simulink model "ad9361_rx_fastattack"  (R2017b)
settings: Solver=ode23  StartTime=0.0  StopTime=inf  RelTol=1e-3  EnableMultiTasking=on
PreLoadFcn:
  | SampleTime_rx = 6.51041666666666667e-8;
  | 
  | adi9361_preload(bdroot,'rx')
undefined symbols (not defined in the file or in its folder): D, dBval, DCLeak_Matrix, fuzz_val, GainImb_Matrix, IP2_Matrix, IP3_Matrix, magnitude, var
libraries: simrfV2elements x13, dsparch4 x8, dspsrcs4 x8, dspmathops x6, dspmlti4 x5, simulink x5, simrfV2util1 x4, fl_lib x4, simrfV2junction1 x3, simulink_extras x2, dspsigattribs x2, simrfV2sources1 x2
(part 1 of 2)
CloseFcn:
  | clear ad9361_rx_hm1Filt ad9361_rx_hm2Filt;
  | clear ad9361_rx_hm3Filt ad9361_rx_hm4Filt;
  | clear SampleTime_rx;
settings Model: SimulationMode=accelerator  Creator=The MathWorks Inc.  LastModifiedBy=ppradhan
settings DataIOCC: ExternalInput=txWaveform  SaveFormat=StructureWithTime  SaveOutput=off  SignalLogging=off  DSMLogging=off  SaveTime=off  OutputSaveName=rx
settings OptimizationCC: DefaultParameterBehavior=Inlined  InlineInvariantSignals=on  EfficientMapNaN2IntZero=off  LifeSpan=inf  SimCompilerOptimization=on
settings DebuggingCC: ReadBeforeWriteMsg=DisableAll  WriteAfterWriteMsg=DisableAll  WriteAfterReadMsg=DisableAll  UnderspecifiedInitializationDetection=Classic  MergeDetectMultiDrivingBlocksExec=none  SolverPrmCheckMsg=warning  InheritedTsInSrcMsg=none  MultiTaskDSMMsg=none  IntegerOverflowMsg=none  AllowSymbolicDim=off  SFUnexpectedBacktrackingDiag=warning  SFNoUnconditionalDefaultTransitionDiag=none  SFUndirectedBroadcastEventsDiag=none  SFExecutionAtInitializationDiag=none  IntegerSaturationMsg=none
settings HardwareCC: ProdBitPerPointer=32  ProdBitPerSizeT=32  ProdBitPerPtrDiffT=32  ProdLargestAtomicFloat=None  ProdIntDivRoundTo=Undefined  ProdEndianess=Unspecified  ProdWordSize=32  ProdHWDeviceType=32-bit Generic  TargetBitPerPointer=64  TargetBitPerSizeT=64  TargetBitPerPtrDiffT=64  TargetLongLongMode=on  TargetIntDivRoundTo=Zero  TargetEndianess=LittleEndian  TargetWordSize=64  TargetHWDeviceType=MATLAB Host  ProdEqTarget=off
settings ModelReferenceCC: UpdateModelReferenceTargets=IfOutOfDate  PropagateSignalLabelsOutOfModel=off
settings SFSimCC: SFSimEcho=off
settings CodeAppCC: MaxIdLength=128  StateflowObjectComments=on
settings GRTTargetCC: TargetLangStandard=C89/C90 (ANSI)  GeneratePreprocessorConditionals=Disable all  CombineOutputUpdateFcns=off  GRTInterface=on
settings ConfigComp: CovMetricSettings=dw  CovHtmlReporting=on  CovSaveCumulativeToWorkspaceVar=on  CovSaveSingleToWorkspaceVar=on  CovExternalEMLEnable=off  CovSFcnEnable=off
settings SimscapeCC: ExplicitSolverDiagnosticOptions=none

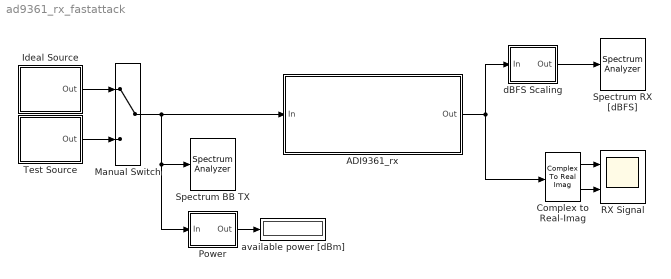
== system ad9361_rx_fastattack ==
  ADI9361_rx : Subsystem  mask(ADI9361_RX){TestSignal=20MHz LTE, LOFreq=2.1e9, Trf=SampleTime_rx/1.5}
      mask prompts: TestSignal "Filter Configuration:"; LOFreq "LO Frequency [Hz]:"; Trf "Step Size RF Simulation [s]:"
      mask help: Model an Analog Devices AD9361 RF Receiver.
      mask init:
      | load ADI9361Tables;
      | ad9361_rx_pars = ad9361_rx_initfcn(gcb,'Init');
      | assignin('base', 'ad9361_rx_hm1Filt', ad9361_rx_pars.ad9361_rx_hm1Filt);
      | assignin('base', 'ad9361_rx_hm2Filt', ad9361_rx_pars.ad9361_rx_hm2Filt);
      | assignin('base', 'ad9361_rx_hm3Filt', ad9361_rx_pars.ad9361_rx_hm3Filt);
      | assignin('base', 'ad9361_rx_hm4Filt', ad9361_rx_pars.ad9361_rx_hm4Filt);
      mask Help:
      | Model an Analog Devices AD9361 RF Receiver. This model predicts thermal noise, spectral growth, LO carrier leakage and image signals, quantization noise in manual and slow attack control mode.
      | 
      | To change the automatic gain control mode, toggle the manual switch between manual mode and slow-attack control mode under the receiver mask. For manual mode, directly specify the index of the gain table in the constant block "manual index".
      | 
      | For signals with LTE 5MHz, LTE 10 MHz and LTE 20 MHz characteristics, the default configurations recommended by Analog Devices are directly available.
      | 
      | The filters are programmable. Use the Analog Devices Wizard App to custom design Filters. Select the option Custom in the Filter Configuration menu and click Design Filter button. The Filter Design app will open automatically. Make sure a receiver filter is designed instead of a transmitter filter. After designing the filter, click the button Export to Workspace in the App. The custom filter design is saved in the model set up. Next time a simulation is setup with custom filter configuration, the latest filter design is used.
      | 
      | Make sure that the input signal sample time and the expected step size of the RF simulation are the same. In case of a mismatch, an error is generated.
      mask TypeOptions TestSignal: 5MHz LTE | 10MHz LTE | 20MHz LTE | Custom
      mask Callback TestSignal:
      | % Set Mask visibilites and enables
      | ad9361_rx_mask_callbacks(gcb,'TestSignal')
      mask DialogControl Control2 Prompt: SpacerDesign
      mask DialogControl DesignFilter Prompt: Design Filter
      mask DialogControl DesignFilter Callback: ad9361_rx_initfcn(gcb,'DesignFilter');
      mask Display: text(0.5,0.5,'AD9361_RX','horizontalAlignment','center');
  Complex to Real-Imag : ComplexToRealImag
  Ideal Source : Subsystem  mask{Sel=Single CW tone, CW=2e6, Pow=-60, Tstep=3.255208333333334e-08, Ovs=1.5}
      mask prompts: Sel "Select source"; CW "Frequency (Hz)"; Pow "Power (dBm)"; Tstep "Sample time (s)"; Ovs "Oversampling"
      mask TypeOptions Sel: CW + 1MHz tone | Single CW tone | Dual CW tone
      mask DialogControl DescGroupVar Prompt: Ideal Test Source
  Manual Switch : ManualSwitch
  "Power  " : Subsystem  mask{R=50}
      mask prompts: R "Reference Impedance [Ohm]"
      mask DialogControl DescGroupVar Prompt: Power Meter
  RX Signal : Scope  NumInputPorts=2
  Spectrum BB TX : SpectrumAnalyzer
  Spectrum RX [dBFS] : SpectrumAnalyzer
  Test Source : Subsystem  mask{TestSigType=20MHz LTE-like test signal, RxCustVector=complex(rand(1000,1), rand(1000,1)), Tstep=3.255208333333334e-08, OverSample=1.5, LTE_Pow=-50, hasBlockerCW=off, CW_Blocker_Freq=3e6, CW_Blocker_Pow=-20, hasBlockerLTE=off, LTE_Blocker_OffsetFreq=3e6, LTE_Blocker_Pow=-30}
      mask prompts: TestSigType "Test signal"; RxCustVector "Custom test vector complex data (I, Q)"; Tstep "Sample time (s)"; OverSample "Oversampling"; LTE_Pow "Power (dBm)"; hasBlockerCW "CW blocker"; CW_Blocker_Freq "Frequency CW blocker (Hz)"; CW_Blocker_Pow "Power CW blocker (dBm)"; hasBlockerLTE "LTE-like blocker"; LTE_Blocker_OffsetFreq "Frequency offset LTE-like blocker (Hz)"; LTE_Blocker_Pow "Power LTE-like blocker (dBm)"
      mask init:
      | load LTE_data;
      | load LTE_blocker;
      | 
      | if strcmpi(TestSigType,'5MHz LTE-like test signal')
      |     tx = tx5;
      |     tx_bl = tx5_bl;
      |     SampleTime_rx = 1/info5.SamplingRate;
      |     LTE = 5;
      | elseif strcmpi(TestSigType,'10MHz LTE-like test signal')
      |     tx = tx10;
      |     tx_bl = tx10_bl;
      |     LTE = 10;
      |     SampleTime_rx = 1/info10.SamplingRate;
      | elseif strcmpi(TestSigType,'20MHz LTE-like test signal')
      |     tx = tx20;
      |     tx_bl = tx20_bl;
      |     LTE = 20;
      |     SampleTime_rx = 1/info20.SamplingRate;
      | elseif strcmpi(TestSigType,'Custom Signal (LTE blocker NOT allowed)')
      |     LTE = 0;
      |     tx = RxCustVector;
      |     tx_bl = RxCustVector;
      |     SampleTime_rx = str2num(get_param(gcb,'Tstep'));
      | else
      |     error(message('simrf:simrfad9361:UnknownTestSig',gcb,TestSigType));
      | end
      | if ~strcmp(TestSigType,'Custom signal (LTE blocker NOT allowed)')
      |     assignin('base', 'SampleTime_rx', SampleTime_rx);
      | end
      | if ~any(strcmpi(get_param(bdroot(gcb), 'SimulationStatus'),             ...
      |         {'running' 'paused'}))
      |     set_param(gcb,'Tstep',num2str(SampleTime_rx,16));
      |     idlSrc = [bdroot '/Ideal Source'];
      |     set_param(idlSrc,'Tstep',num2str(SampleTime_rx,16));
      |     p = Simulink.Mask.get(gcb);
      |     p.Parameters(3).Value = num2str(SampleTime_rx,16);
      | end
      mask TypeOptions TestSigType: 5MHz LTE-like test signal | 10MHz LTE-like test signal | 20MHz LTE-like test signal | Custom Signal (LTE blocker NOT allowed)
      mask Callback TestSigType:
      | % Set Mask visibilites and enables
      | ad9361_rx_mask_callbacks(gcb,'TestSigType')
      mask Callback hasBlockerCW:
      | % Set Mask visibilites and enables
      | ad9361_rx_mask_callbacks(gcb,'hasBlockerCW')
      mask Callback hasBlockerLTE:
      | % Set Mask visibilites and enables
      | ad9361_rx_mask_callbacks(gcb,'hasBlockerLTE')
      mask DialogControl DescGroupVar Prompt: Test Source RX
  available power [dBm] : Display
  dBFS Scaling : Subsystem
  wires:
  Test Source/1(Out) -> Manual Switch/2
  Ideal Source/1(Out) -> Manual Switch/1
  Manual Switch/1 -> Spectrum BB TX/1, "Power  "/1(In), ADI9361_rx/1(In)
  "Power  "/1(Out) -> available power [dBm]/1
  dBFS Scaling/1(Out) -> Spectrum RX [dBFS]/1
  ADI9361_rx/1(Out) -> Complex to Real-Imag/1, dBFS Scaling/1(In)
  Complex to Real-Imag/1 -> RX Signal/1
  Complex to Real-Imag/2 -> RX Signal/2

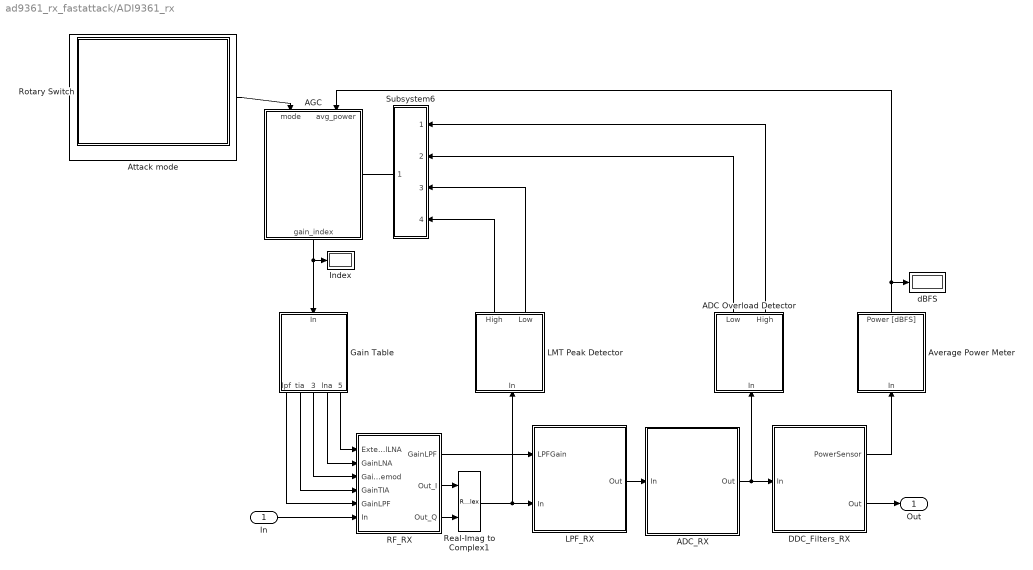
== system ad9361_rx_fastattack/ADI9361_rx ==
  In : Inport
  ADC Overload Detector : Subsystem  mask{Ncycles=4, Lthreshold=47, Hthreshold=58}
      mask prompts: Ncycles "Number of Integration Cycles"; Lthreshold "Low Threshold"; Hthreshold "High Threshold"
      mask DialogControl DescGroupVar Prompt: ADC Overload Detector
  ADC_RX : Subsystem
  AGC : Stateflow chart  TreatAsAtomicUnit=on  mask{T=1, PeakOverLoadWait=1, SettlingDelay=32, FIR_Ts=ad9361_rx_pars.Tadc*ad9361_rx_pars.HB_interp, LMT_G_dec_fast=2, ADC_G_dec_fast=2, AGC_G_dec_fast=1, AGC_G_dec_slow=1, AGC_G_inc_fast=1, AGC_G_inc_slow=1, ManualGainIndex=76, C=61440 %approx 1ms, N_LMT_H=10, N_LMT_L=10, N_ADC_H=10, N_ADC_L=10, PT_HH=-8, PT_H=-10, PT_L=-12, PT_LL=-15, AGC_lock_level=-10, Max_Increase=5, EnableIncrGain=1, EnableGainIncAfterLock=1, AGC_attack_delay=10, EnergyDetectCount=32, IncrTime=5, LowPower=-13, PostLockStepSize=1, PowerMeasDuration=64, GainReset=Max Gain, GainOffset=5, EnergyLost=1, StrongerSignalThreshold=10, GainLockExitCount=8, Overrange=8}
      mask prompts: T "Extra delay margin [us]"; PeakOverLoadWait "Peak Overload Wait Time [cycles]"; SettlingDelay "Settling Delay Power Meter [cycles]"; FIR_Ts "FIR Input Clock Time"; LMT_G_dec_fast "LMT peak large decrement"; ADC_G_dec_fast "ADC peak large decrement"; AGC_G_dec_fast "Average Power large decrement"; AGC_G_dec_slow "Average Power small decrement"; AGC_G_inc_fast "Average Power large increment"; AGC_G_inc_slow "Average Power small increment"; ManualGainIndex "Gain Index"; C "Gain Update Counter [cycles]"; N_LMT_H "LMT Upper Count"; N_LMT_L "LMT Lower Count"; N_ADC_H "ADC Upper Count"; N_ADC_L "ADC Lower Count"; PT_HH "Outer Threshold High [dBFS]"; PT_H "Inner Threshold High [dBFS]"; PT_L "Inner Threshold Low [dBFS]"; PT_LL "Outer Threshold Low [dBFS]"; AGC_lock_level "AGC Lock Level [dBFS]"; Max_Increase "AGC Lock Level Max Increase [Index]"; EnableIncrGain "Enable Gain Increment [0/1]"; EnableGainIncAfterLock "Enable Gain Increment After Gain Lock [0/1]"; AGC_attack_delay "Attack delay [us]"; EnergyDetectCount "Energy Detect Count [cycles]"; IncrTime "Increment Time [cycles]"; LowPower "Low Power Threshold"; PostLockStepSize "Post Lock Level Step Size [Index]"; PowerMeasDuration "Power Measurement Duration - State 5 [cycles]"; GainReset "Gain Index When Reset"; GainOffset "Optimize Gain Offset"; EnergyLost "Energy Lost Level [dB]"; StrongerSignalThreshold "Stronger Signal Threshold [dB]"; GainLockExitCount "Gain Lock Exit Count [cycles]"; Overrange "Overrange Count [Events]"
      mask init:
      | EnergyDetectCount = EnergyDetectCount*FIR_Ts;
      | C = C*FIR_Ts;
      | SettlingDelay = SettlingDelay*FIR_Ts;
      | PeakOverLoadWait = PeakOverLoadWait*FIR_Ts;
      | PowerMeasDuration = PowerMeasDuration*FIR_Ts;
      | IncrTime = IncrTime*FIR_Ts;
      | 
      | tmp = get_param(gcb,'parent');
      | n = get_param([tmp, '/Average Power Meter'], 'Ncycles');
      | DecPowerMeasDuration = str2num(n)*FIR_Ts;
  Attack mode : Constant  Value=0  SampleTime=-1
  Average Power Meter : Subsystem  mask{Ncycles=64}
      mask prompts: Ncycles "Number of Integration Cycles"
      mask DialogControl DescGroupVar Prompt: Average Power Meter
  DDC_Filters_RX : Subsystem
  Gain Table : Subsystem
  "Index " : Display
  LMT Peak Detector : Subsystem  mask{HThreshold=800, LThreshold=704}
      mask prompts: HThreshold "High Threshold [mV]"; LThreshold "Low Threshold [mV]"
      mask DialogControl DescGroupVar Prompt: LMT Peak Detector
  LPF_RX : Subsystem
  RF_RX : Subsystem  mask{RF=LOFreq, Tstep=Trf, Imp=on}
      mask prompts: RF "Center Frequency [Hz]"; Tstep "Sample Time [s]"; Imp "RF Impairments [on/off]"
      mask init:
      | freq = [0.8e9, 2.4e9, 5.5e9];
      | nf   = [2,       3,        3.8];
      | NF   = interp1(freq, nf, RF);
      | 
      | index_gain3  = [6,  16, 20, 23, 28,  30,  33, 34, 36, 37, 54, 55,  73,  76];
      | iip3_800MHz  = [10, 10, 10, 8,   8,   10,  9,   -3, -5, -5, -8, -13, -14, -18];
      | iip3_2p4GHz  = [9,  9,   9,   8,   7,    9,   8,   0,   0,  -5, -5, -7,   -8,   -10];
      | iip3_5p5GHz  = [16,10, 10, 11,  11, 11, 11,  11, 11, -3, -6, -7,  -10, -16];
      | 
      | index_gain2  = [20, 36, 68, 76];
      | iip2_800MHz  = [80, 80, 58, 48];
      | iip2_2p4GHz  = [70, 70, 60, 50];
      | iip2_5p5GHz  = [70, 70, 60, 45];
      | 
      | if RF<=1.3e9
      |     ind_lna = (0:3);
      |     lna_gain = [5, 17, 19 24];
      |     ind_mixer = (0:15);
      |     mixer_gain = [0, 3, 9, (2:14)+11];
      |     ind_tia = (0:1);
      |     tia_gain = [-6, 0];
      |     IIP3 = iip3_800MHz;
      |     IIP2 = iip2_800MHz;
      | elseif RF <= 4e9
      |     ind_lna = (0:3);
      |     lna_gain = [3, 14, 17, 21];
      |     ind_mixer = (0:15);
      |     mixer_gain = [0, 3, 9, (3:15)+11];
      |     ind_tia = (0:1);
      |     tia_gain = [-6, 0];
      |     IIP3 = iip3_2p4GHz;
      |     IIP2 = iip2_2p4GHz;
      | else
      |     ind_lna = (0:3);
      |     lna_gain = [-4, 10, 13, 14];
      |     ind_mixer = (0:15);
      |     mixer_gain = [0, 3, 8, (1:13)+11];
      |     ind_tia = (0:1);
      |     tia_gain = [-6, 0];
      |     IIP3 = iip3_5p5GHz;
      |     IIP2 = iip2_5p5GHz;
      | end
      | %index = [0 16 26 36 46 56 66 76];
      | index  = [0 6 15 26 37 48 58 69 76];
      | if Imp == 0
      |     NF = 0;
      |     IIP3 = 500*ones(1,14);
      |     IIP2 = 500*ones(1,4);
      |     Rin = 50;
      |     set_param([gcb '/Configuration'], 'AddNoise','off'); 
      |     gainImbalance = -500*ones(size(index));
      |     DCleak = -500*ones(size(index));
      |     disp('Ideal RF receiver')
      | else
      |     S11 = -200;
      |     Rin = s2z(10^(S11/20));
      |     set_param([gcb '/Configuration'], 'AddNoise','on');
      |     %index        = [0     6  15  26  37  48  58  69  76];
      |     DCleak        = [-66 -72 -72 -74 -69 -70 -69 -71 -68]-5;
      |     gainImbalance = [-80 -75 -79 -82 -83 -82 -79 -73 -65]+10;
      |     %gainImbalance = [-85   -87.5 -89.5 -89   -88.5 -88   -80   -72]; 
      |     %DCleak        = [-80.5 -92.5 -93.5 -83.5 -85   -82.5 -86   -79];
      | end
      mask DialogControl DescGroupVar Prompt: ADI 9361 Receiver RF Parameters
  Real-Imag to Complex1 : RealImagToComplex
  Rotary Switch : Subsystem  DialogController=hmiCreateDDGDialog  IsWebBlock=on  mask(MWDashboardBlock){webBlockId=b4c78a3e-b6a7-4745-80e9-7b467905a983, webBlockType=discreteknob, ShowInLibBrowser=on, ShowInitialText=on, HMISrcModelName=ad9361_rx_fastattack}
      mask prompts: webBlockId "WebBlock Id"; webBlockType "WebBlock Type"; HMISrcModelName "Source Model"
      mask Help: helpview([docroot '/mapfiles/simulink.map'], 'hmi_rotary_switch')
      mask Display:
      | model = bdroot(gcb);
      | if strcmp(get_param(model,'BlockDiagramType'), 'library')
      |     image([(matlabroot) '/toolbox/simulink/hmi/icons/DiscreteKnob.png']);
      | end
  Subsystem6 : Subsystem  mask{NCyclesADC=4}
      mask prompts: NCyclesADC "ADC Integration Cycles"
  dBFS : Display
  Out : Outport
  wires:
  RF_RX/2(Out_I) -> Real-Imag to Complex1/1
  RF_RX/3(Out_Q) -> Real-Imag to Complex1/2
  Real-Imag to Complex1/1 -> LMT Peak Detector/1(In), LPF_RX/2(In)
  Gain Table/2(tia) -> RF_RX/4(GainTIA)
  Gain Table/3(demod) -> RF_RX/3(GainDemod)
  Gain Table/4(lna) -> RF_RX/2(GainLNA)
  LPF_RX/1(Out) -> ADC_RX/1(In)
  LMT Peak Detector/2(Low) -> Subsystem6/3(LMT_L)
  Gain Table/1(lpf) -> RF_RX/5(GainLPF)
  DDC_Filters_RX/1(PowerSensor) -> Average Power Meter/1(In)
  ADC Overload Detector/2(High) -> Subsystem6/1(ADC_H)
  LMT Peak Detector/1(High) -> Subsystem6/4(LMT_H)
  ADC Overload Detector/1(Low) -> Subsystem6/2(ADC_L)
  DDC_Filters_RX/2(Out) -> Out/1
  In/1 -> RF_RX/6(In)
  Subsystem6/1(Peak) -> AGC/Trigger
  RF_RX/1("GainLPF ") -> LPF_RX/1(LPFGain)
  Gain Table/5(External LNA) -> RF_RX/1(ExternalLNA)
  Attack mode/1 -> AGC/1(mode)
  Average Power Meter/1(Power [dBFS]) -> dBFS/1, AGC/2(avg_power)
  AGC/1(gain_index) -> "Index "/1, Gain Table/1(In)
  ADC_RX/1(Out) -> ADC Overload Detector/1(In), DDC_Filters_RX/1(In)

== system ad9361_rx_fastattack/Ideal Source ==
  2Tones : dspsrcs4/Sine Wave  Amplitude=sqrt(2)  Frequency=CW/2  Phase=0  SampleMode=Discrete  OutComplex=Real  CompMethod=Trigonometric fcn  TableSize=Speed  SampleTime=Tstep/Ovs  SamplesPerFrame=1  ResetState=Restart at time zero  OutputFrames=on  dataType=double  wordLen=16  udDataType=sfix(16)  fracBitsMode=Best precision  numFracBits=15  OutDataTypeStr=double  LastOutDataTypeStr=double
  CW : dspsrcs4/Sine Wave  Amplitude=1  Frequency=CW  Phase=0  SampleMode=Discrete  OutComplex=Complex  CompMethod=Trigonometric fcn  TableSize=Speed  SampleTime=Tstep/Ovs  SamplesPerFrame=1  ResetState=Restart at time zero  OutputFrames=on  dataType=double  wordLen=16  udDataType=sfix(16)  fracBitsMode=Best precision  numFracBits=15  OutDataTypeStr=double  LastOutDataTypeStr=double
  CW+Modulation : dspsrcs4/Sine Wave  Amplitude=[1; 1]/sqrt(2)  Frequency=[CW; 1e6]  Phase=[0; 0]  SampleMode=Discrete  OutComplex=Complex  CompMethod=Trigonometric fcn  TableSize=Speed  SampleTime=Tstep/Ovs  SamplesPerFrame=1  ResetState=Restart at time zero  OutputFrames=on  dataType=double  wordLen=16  udDataType=sfix(16)  fracBitsMode=Best precision  numFracBits=15  OutDataTypeStr=double  LastOutDataTypeStr=double
  Constant : Constant  Value=Sel  SampleTime=Tstep/Ovs
  Multiport Switch : MultiPortSwitch
  Real-Imag to Complex : RealImagToComplex  Input=Real
  Sum of Elements : Sum  Inputs=+
  dB Gain : dspmathops/dB Gain  dB=Pow-30+20*log10(sqrt(50))  intype=Amplitude
      settings: SourceProductName=DSP System Toolbox  SourceProductBaseCode=DS
  Out : Outport
  wires:
  dB Gain/1 -> Out/1
  Multiport Switch/1 -> dB Gain/1
  Real-Imag to Complex/1 -> Multiport Switch/4
  Constant/1 -> Multiport Switch/1
  2Tones/1 -> Real-Imag to Complex/1
  CW/1 -> Multiport Switch/3
  Sum of Elements/1 -> Multiport Switch/2
  CW+Modulation/1 -> Sum of Elements/1

== system ad9361_rx_fastattack/Power   ==
  In : Inport
  CountNCycles : Buffer  N=1024
  Frame Conversion : FrameConversion  InheritSamplingMode=off  OutFrame=Sample-based
  Gain2 : Gain  Gain=1/1024
  Root : Sqrt  SaturateOnIntegerOverflow=on
  Squared : Math  Operator=magnitude^2  SaturateOnIntegerOverflow=on
  Sum : Sum  Inputs=+
  dB Conversion : dspmathops/dB Conversion  dBtype=dBm  intype=Amplitude  R=R  fuzz=on
      settings: SourceProductName=DSP System Toolbox
  Out : Outport
  wires:
  dB Conversion/1 -> Out/1
  In/1 -> CountNCycles/1
  Frame Conversion/1 -> dB Conversion/1
  CountNCycles/1 -> Squared/1
  Squared/1 -> Sum/1
  Sum/1 -> Gain2/1
  Root/1 -> Frame Conversion/1
  Gain2/1 -> Root/1

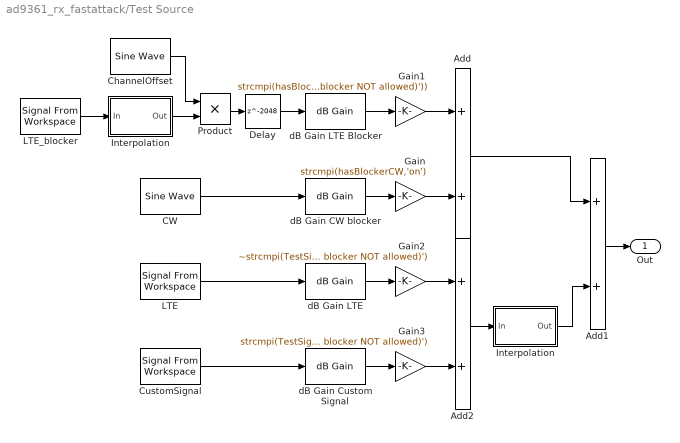
== system ad9361_rx_fastattack/Test Source ==
  Add : Sum
  Add1 : Sum
  Add2 : Sum
  CW : dspsrcs4/Sine Wave  Amplitude=1  Frequency=CW_Blocker_Freq  Phase=0  SampleMode=Discrete  OutComplex=Complex  CompMethod=Trigonometric fcn  TableSize=Speed  SampleTime=Tstep/OverSample  SamplesPerFrame=1  ResetState=Restart at time zero  OutputFrames=on  dataType=double  wordLen=16  udDataType=sfix(16)  fracBitsMode=Best precision  numFracBits=15  OutDataTypeStr=double  LastOutDataTypeStr=double
  ChannelOffset : dspsrcs4/Sine Wave  Amplitude=1  Frequency=LTE_Blocker_OffsetFreq  Phase=0  SampleMode=Discrete  OutComplex=Complex  CompMethod=Trigonometric fcn  TableSize=Speed  SampleTime=Tstep/OverSample  SamplesPerFrame=1  ResetState=Restart at time zero  OutputFrames=on  dataType=double  wordLen=16  udDataType=sfix(16)  fracBitsMode=Best precision  numFracBits=15  OutDataTypeStr=double  LastOutDataTypeStr=double
  CustomSignal : dspsrcs4/Signal From Workspace  X=repmat(tx,10,1)  Ts=Tstep  nsamps=1  OutputAfterFinalValue=Setting to zero  ignoreOrWarnInputAndFrameLengths=off  OutputFrames=on
  Delay : Delay  DelayLength=2048
  Gain : Gain  Gain=strcmpi(hasBlockerCW,'on')
  Gain1 : Gain  Gain=strcmpi(hasBlockerLTE,'on')&&(~strcmpi(TestSigType,'Custom Signal (LTE blocker NOT allowed)'))
  Gain2 : Gain  Gain=~strcmpi(TestSigType,'Custom Signal (LTE blocker NOT allowed)')
  Gain3 : Gain  Gain=strcmpi(TestSigType,'Custom Signal (LTE blocker NOT allowed)')
  Interpolation : Subsystem
  "Interpolation " : Subsystem
  LTE : dspsrcs4/Signal From Workspace  X=repmat(tx,10,1)  Ts=Tstep  nsamps=1  OutputAfterFinalValue=Setting to zero  ignoreOrWarnInputAndFrameLengths=off  OutputFrames=on
  LTE_blocker : dspsrcs4/Signal From Workspace  X=repmat(tx_bl,10,1)  Ts=Tstep  nsamps=1  OutputAfterFinalValue=Setting to zero  ignoreOrWarnInputAndFrameLengths=off  OutputFrames=on
  Product : Product
  dB Gain CW blocker : dspmathops/dB Gain  dB=CW_Blocker_Pow-30+20*log10(sqrt(50))  intype=Amplitude
      settings: SourceProductName=DSP System Toolbox  SourceProductBaseCode=DS
  dB Gain Custom Signal : dspmathops/dB Gain  dB=LTE_Pow - (10*log10(var(tx))+30)+20*log10(sqrt(50))  intype=Amplitude
      settings: SourceProductName=DSP System Toolbox  SourceProductBaseCode=DS
  dB Gain LTE : dspmathops/dB Gain  dB=LTE_Pow-10*log10(var(tx))-12  intype=Amplitude
      settings: SourceProductName=DSP System Toolbox  SourceProductBaseCode=DS
  dB Gain LTE Blocker : dspmathops/dB Gain  dB=LTE_Blocker_Pow-10*log10(var(tx_bl))-12  intype=Amplitude
      settings: SourceProductName=DSP System Toolbox  SourceProductBaseCode=DS
  Out : Outport
  wires:
  dB Gain CW blocker/1 -> Gain/1
  Gain/1 -> Add/2
  LTE/1 -> dB Gain LTE/1
  LTE_blocker/1 -> Interpolation/1(In)
  Gain1/1 -> Add/1
  Interpolation/1(Out) -> Product/2
  Product/1 -> Delay/1
  ChannelOffset/1 -> Product/1
  dB Gain LTE/1 -> Gain2/1
  dB Gain LTE Blocker/1 -> Gain1/1
  Gain2/1 -> Add2/1
  dB Gain Custom Signal/1 -> Gain3/1
  Gain3/1 -> Add2/2
  Delay/1 -> dB Gain LTE Blocker/1
  CustomSignal/1 -> dB Gain Custom Signal/1
  Add2/1 -> "Interpolation "/1(In)
  Add/1 -> Add1/1
  "Interpolation "/1(Out) -> Add1/2
  Add1/1 -> Out/1
  CW/1 -> dB Gain CW blocker/1

== system ad9361_rx_fastattack/dBFS Scaling ==
  In : Inport
  Gain : Gain  Gain=1/2047
  Out : Outport
  wires:
  In/1 -> Gain/1
  Gain/1 -> Out/1

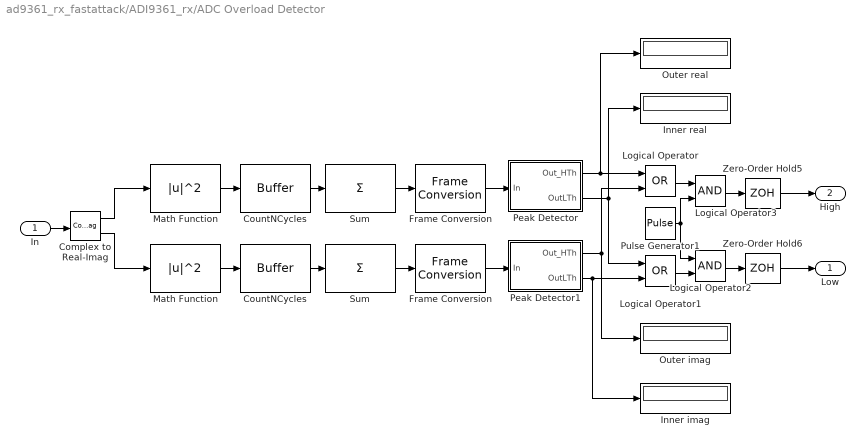
== system ad9361_rx_fastattack/ADI9361_rx/ADC Overload Detector ==
  In : Inport
  Complex to Real-Imag : ComplexToRealImag
  CountNCycles : Buffer  N=Ncycles
  "CountNCycles " : Buffer  N=Ncycles
  Frame Conversion : FrameConversion  InheritSamplingMode=off  OutFrame=Sample-based
  "Frame Conversion " : FrameConversion  InheritSamplingMode=off  OutFrame=Sample-based
  Inner imag : Display
  Inner real : Display
  Logical Operator : Logic  Operator=OR  AllPortsSameDT=off  OutDataTypeStr=boolean
  Logical Operator1 : Logic  Operator=OR  AllPortsSameDT=off  OutDataTypeStr=boolean
  Logical Operator2 : Logic  AllPortsSameDT=off  OutDataTypeStr=boolean
  Logical Operator3 : Logic  AllPortsSameDT=off  OutDataTypeStr=boolean
  Math Function : Math  Operator=magnitude^2  SaturateOnIntegerOverflow=on
  "Math Function " : Math  Operator=magnitude^2  SaturateOnIntegerOverflow=on
  Outer imag : Display
  Outer real : Display
  Peak Detector : Subsystem  mask{HThreshold=Hthreshold, LThreshold=Lthreshold}
      mask prompts: HThreshold "High Threshold (bit string) <4:0>"; LThreshold "Low Threshold (bit string) <4:0>"
  Peak Detector1 : Subsystem  mask{HThreshold=Hthreshold, LThreshold=Lthreshold}
      mask prompts: HThreshold "High Threshold (bit string) <4:0>"; LThreshold "Low Threshold (bit string) <4:0>"
  Pulse Generator1 : DiscretePulseGenerator  SampleTime=ad9361_rx_pars.Tadc*Ncycles
  Sum : Sum  Inputs=+
  "Sum " : Sum  Inputs=+
  Zero-Order Hold5 : ZeroOrderHold  SampleTime=Trf
  Zero-Order Hold6 : ZeroOrderHold  SampleTime=Trf
  Low : Outport
  High : Outport  Port=2
  wires:
  Math Function/1 -> CountNCycles/1
  CountNCycles/1 -> Sum/1
  Sum/1 -> Frame Conversion/1
  Frame Conversion/1 -> Peak Detector/1(In)
  In/1 -> Complex to Real-Imag/1
  "Math Function "/1 -> "CountNCycles "/1
  "CountNCycles "/1 -> "Sum "/1
  "Sum "/1 -> "Frame Conversion "/1
  "Frame Conversion "/1 -> Peak Detector1/1(In)
  Peak Detector/2(OutLTh) -> Logical Operator1/1, Inner real/1
  Peak Detector/1(Out_HTh) -> Outer real/1, Logical Operator/1
  Peak Detector1/1(Out_HTh) -> Logical Operator/2, Outer imag/1
  Peak Detector1/2(OutLTh) -> Inner imag/1, Logical Operator1/2
  Complex to Real-Imag/1 -> Math Function/1
  Complex to Real-Imag/2 -> "Math Function "/1
  Logical Operator/1 -> Logical Operator3/1
  Logical Operator2/1 -> Zero-Order Hold6/1
  Logical Operator1/1 -> Logical Operator2/2
  Logical Operator3/1 -> Zero-Order Hold5/1
  Pulse Generator1/1 -> Logical Operator2/1, Logical Operator3/2
  Zero-Order Hold5/1 -> High/1
  Zero-Order Hold6/1 -> Low/1

== system ad9361_rx_fastattack/ADI9361_rx/ADC_RX ==
  In : Inport
  ADC_I : Subsystem
  ADC_Q : Subsystem
  Complex to Real-Imag1 : ComplexToRealImag
  Real-Imag to Complex : RealImagToComplex
  Out : Outport
  wires:
  Complex to Real-Imag1/1 -> ADC_I/1(In)
  Complex to Real-Imag1/2 -> ADC_Q/1(In)
  In/1 -> Complex to Real-Imag1/1
  Real-Imag to Complex/1 -> Out/1
  ADC_I/1(Out) -> Real-Imag to Complex/1
  ADC_Q/1(Out) -> Real-Imag to Complex/2

== system ad9361_rx_fastattack/ADI9361_rx/Average Power Meter ==
  In : Inport
  Max saturation power dBm : Constant  Value=20*log10(4)+30
  Quantizer : Quantizer
  RMS : Subsystem
  Saturation : Saturate  UpperLimit=0  LowerLimit=-63.5
  Subtract : Sum  Inputs=+-
  dB Conversion : Subsystem  mask(dB Conversion){dBtype=dBm, intype=Amplitude, R=1, fuzz=on}
      mask prompts: dBtype "Convert to:"; intype "Input signal:"; R "Load resistance (ohms):"; fuzz "Add eps to input to protect against  "log(0) = -inf""
      mask help: Convert input of watts or volts to decibels. Voltage inputs are first converted to power relative to the specified load resistance, where P = (V^2)/R. When converting to dB, the reference power is 1 W. When converting to dBm, the reference power is 1 mW.
      mask init:
      | [str fuzz_val dBval] = dspblkdb2('init');
      | dspblkdb2('checkparam');
      | dspblkdb2('update');
      mask Help: eval('blocksethelp');
      mask TypeOptions dBtype: dB | dBm
      mask Callback dBtype: dspblkdb2
      mask TypeOptions intype: Power | Amplitude
      mask Callback intype: dspblkdb2
      mask Display: disp(str)
  Power [dBFS] : Outport
  wires:
  Max saturation power dBm/1 -> Subtract/2
  Subtract/1 -> Quantizer/1
  Quantizer/1 -> Saturation/1
  dB Conversion/1(out) -> Subtract/1
  In/1 -> RMS/1(In)
  RMS/1(Out) -> dB Conversion/1(in)
  Saturation/1 -> Power [dBFS]/1

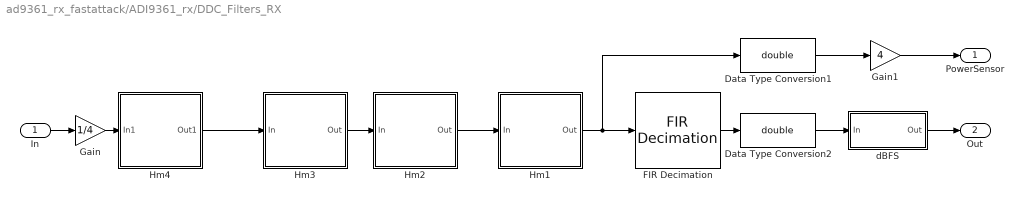
== system ad9361_rx_fastattack/ADI9361_rx/DDC_Filters_RX ==
  In : Inport
  Data Type Conversion1 : DataTypeConversion  OutDataTypeStr=double
  Data Type Conversion2 : DataTypeConversion  OutDataTypeStr=double
  FIR Decimation : dspmlti4/FIR Decimation  FilterSource=Filter object  h=fir1(35,0.4)  D=2  filtStruct=Direct form  FilterObject=ad9361_rx_pars.Hmd_rx  framing=Allow multirate processing  inputOffset=0  outputBufInitCond=0  roundingMode=Floor  overflowMode=off  firstCoeffDataTypeStr=Inherit: Same word length as input  firstCoeffMin=[]  firstCoeffMax=[]  firstCoeffLastDataTypeStr=Inherit: Same word length as input  outputDataTypeStr=Inherit: Same as accumulator  outputMin=[]  outputMax=[]  outputLastDataTypeStr=Inherit: Same as accumulator
  Gain : Gain  Gain=1/4
  Gain1 : Gain  Gain=4
  Hm1 : Subsystem  Variant=on
  Hm2 : Subsystem  Variant=on
  Hm3 : Subsystem  Variant=on
  Hm4 : Subsystem  Variant=on
  dBFS : Subsystem
  PowerSensor : Outport
  Out : Outport  Port=2
  wires:
  In/1 -> Gain/1
  Hm4/1(Out1) -> Hm3/1(In)
  Hm3/1(Out) -> Hm2/1(In)
  Hm2/1(Out) -> Hm1/1(In)
  FIR Decimation/1 -> Data Type Conversion2/1
  Gain/1 -> Hm4/1(In1)
  Data Type Conversion1/1 -> Gain1/1
  Gain1/1 -> PowerSensor/1
  Hm1/1(Out) -> FIR Decimation/1, Data Type Conversion1/1
  Data Type Conversion2/1 -> dBFS/1(In)
  dBFS/1(Out) -> Out/1

== system ad9361_rx_fastattack/ADI9361_rx/Gain Table ==
  In : Inport
  Delay1 : Delay  DelayLength=1  InitialCondition=76  SampleTime=Trf
  Demux : Demux  Outputs=6
  Direct Lookup Table (n-D) : LookupNDDirect  InputsSelectThisObjectFromTable=Column  Table=ADIGainTable'
  Index : Terminator
  lpf : Outport
  tia : Outport  Port=2
  demod : Outport  Port=3
  lna : Outport  Port=4
  External LNA : Outport  Port=5
  wires:
  Demux/3 -> demod/1
  Demux/2 -> lna/1
  Demux/4 -> tia/1
  Demux/5 -> lpf/1
  In/1 -> Delay1/1
  Delay1/1 -> Direct Lookup Table (n-D)/1
  Direct Lookup Table (n-D)/1 -> Demux/1
  Demux/6 -> External LNA/1
  Demux/1 -> Index/1

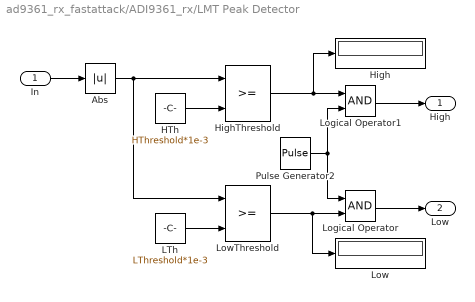
== system ad9361_rx_fastattack/ADI9361_rx/LMT Peak Detector ==
  In : Inport
  Abs : Abs
  HTh : Constant  Value=HThreshold*1e-3
  "High " : Display
  HighThreshold : RelationalOperator  OutDataTypeStr=boolean  RndMeth=Nearest
  LTh : Constant  Value=LThreshold*1e-3
  Logical Operator : Logic  AllPortsSameDT=off  OutDataTypeStr=boolean
  Logical Operator1 : Logic  AllPortsSameDT=off  OutDataTypeStr=boolean
  "Low " : Display
  LowThreshold : RelationalOperator  OutDataTypeStr=boolean  RndMeth=Nearest
  Pulse Generator2 : DiscretePulseGenerator  SampleTime=Trf
  High : Outport  SampleTime=Trf
  Low : Outport  Port=2  SampleTime=Trf
  wires:
  LTh/1 -> LowThreshold/2
  Abs/1 -> HighThreshold/1, LowThreshold/1
  HTh/1 -> HighThreshold/2
  In/1 -> Abs/1
  HighThreshold/1 -> Logical Operator1/1, "High "/1
  LowThreshold/1 -> Logical Operator/2, "Low "/1
  Pulse Generator2/1 -> Logical Operator1/2, Logical Operator/1
  Logical Operator1/1 -> High/1
  Logical Operator/1 -> Low/1

== system ad9361_rx_fastattack/ADI9361_rx/LPF_RX ==
  LPFGain : Inport
  In : Inport  Port=2
  AntiAliasing : dsparch4/Analog Filter Design  method=Butterworth  filttype=Lowpass  N=3  Wlo=1.4*ad9361_rx_pars.Fpass*2*pi  Whi=80  Rp=2  Rs=40
  "AntiAliasing " : dsparch4/Analog Filter Design  method=Butterworth  filttype=Lowpass  N=3  Wlo=1.4*ad9361_rx_pars.Fpass*2*pi  Whi=80  Rp=2  Rs=40
  Complex to Real-Imag : ComplexToRealImag
  Gain : Product
  Real-Imag to Complex1 : RealImagToComplex
  dB2lin : Subsystem
  Out : Outport
  wires:
  Complex to Real-Imag/1 -> AntiAliasing/1
  Real-Imag to Complex1/1 -> Out/1
  In/1 -> Gain/2
  LPFGain/1 -> dB2lin/1(In)
  Gain/1 -> Complex to Real-Imag/1
  dB2lin/1(Out) -> Gain/1
  "AntiAliasing "/1 -> Real-Imag to Complex1/2
  AntiAliasing/1 -> Real-Imag to Complex1/1
  Complex to Real-Imag/2 -> "AntiAliasing "/1

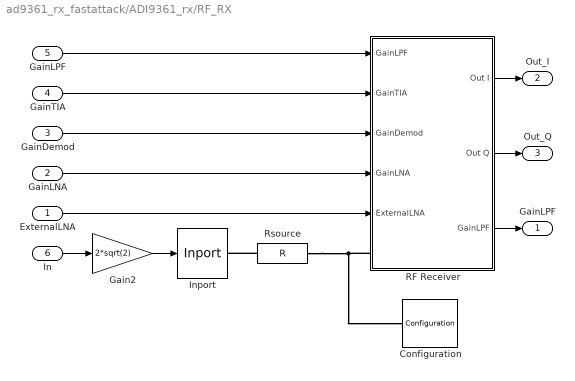
== system ad9361_rx_fastattack/ADI9361_rx/RF_RX ==
  ExternalLNA : Inport
  GainLNA : Inport  Port=2
  GainDemod : Inport  Port=3
  GainTIA : Inport  Port=4
  GainLPF : Inport  Port=5
  In : Inport  Port=6
  Configuration : simrfV2util1/Configuration  AutoFreq=off  Tones=RF Hz  Harmonics=3  NormalizeCarrierPower=on  SolverType=Auto  StepSize=Tstep s  AddNoise=on  defaultRNG=on  Seed=0  Temperature=290.0 K  SolverDelFlag=0
      settings: SourceProductName=RF Blockset  SourceProductBaseCode=RB
  Gain2 : Gain  Gain=2*sqrt(2)
  Inport : simrfV2util1/Inport  SimulinkInputSignalType=Ideal voltage  CarrierFreq=RF Hz  ZS=0  InternalGrounding=on
      settings: SourceProductName=RF Blockset  SourceProductBaseCode=RB
  RF Receiver : Subsystem
  Rsource : simrfV2elements/R  classname=resistor  Resistance=50 Ohm  AddNoise=on
      settings: SourceProductName=RF Blockset  SourceProductBaseCode=RB
  "GainLPF " : Outport
  Out_I : Outport  Port=2
  Out_Q : Outport  Port=3
  wires:
  In/1 -> Gain2/1
  GainTIA/1 -> RF Receiver/2(GainTIA)
  GainDemod/1 -> RF Receiver/3(GainDemod)
  GainLNA/1 -> RF Receiver/4(GainLNA)
  GainLPF/1 -> RF Receiver/1(GainLPF)
  Gain2/1 -> Inport/1
  RF Receiver/1(Out I) -> Out_I/1
  RF Receiver/2(Out Q) -> Out_Q/1
  RF Receiver/3("GainLPF ") -> "GainLPF "/1
  ExternalLNA/1 -> RF Receiver/5(ExternalLNA)
  connections:
  RF Receiver/LConn1 -- Rsource/LConn1 -- Configuration/LConn1
  Rsource/RConn1 -- Inport/RConn1

== system ad9361_rx_fastattack/ADI9361_rx/Rotary Switch ==

== system ad9361_rx_fastattack/ADI9361_rx/Subsystem6 ==
  ADC_H : Inport
  ADC_L : Inport  Port=2
  LMT_L : Inport  Port=3
  LMT_H : Inport  Port=4
  Data Type Conversion : DataTypeConversion  OutDataTypeStr=boolean
  Logical Operator : Logic  Operator=OR  AllPortsSameDT=off  OutDataTypeStr=boolean
  Mux : Mux  Inputs=5
  Subsystem1 : Subsystem
  Wblk5 : Subsystem
  Wblk6 : Subsystem
  Wblk7 : Subsystem
  Peak : Outport
  wires:
  LMT_L/1 -> Wblk7/1(Win)
  Logical Operator/1 -> Wblk7/2(Sin), Wblk6/2(Sin)
  Wblk7/1(Wout) -> Mux/3  "LMT_L"
  Wblk6/1(Wout) -> Mux/2  "ADC_L"
  Wblk5/1(Wout) -> Mux/1, Logical Operator/1  "ADC_H"
  Subsystem1/1(START) -> Data Type Conversion/1
  Data Type Conversion/1 -> Mux/5  "Event"
  ADC_L/1 -> Wblk6/1(Win)
  ADC_H/1 -> Wblk5/1(Win)
  LMT_H/1 -> Wblk5/2(Sin), Mux/4, Logical Operator/2  "LMT_H"
  Mux/1 -> Peak/1

== system ad9361_rx_fastattack/Test Source/Interpolation ==
  In : Inport
  AntiAliasing : dsparch4/Analog Filter Design  method=Elliptic  filttype=Lowpass  N=8  Wlo=2*pi/(2*Tstep)  Whi=80  Rp=0.1  Rs=80
  "AntiAliasing " : dsparch4/Analog Filter Design  method=Elliptic  filttype=Lowpass  N=8  Wlo=2*pi/(2*Tstep)  Whi=80  Rp=0.1  Rs=80
  Complex to Real-Imag : ComplexToRealImag
  Real-Imag to Complex1 : RealImagToComplex
  Zero-Order Hold : ZeroOrderHold  SampleTime=Tstep/OverSample
  "Zero-Order Hold " : ZeroOrderHold  SampleTime=Tstep/OverSample
  Out : Outport
  wires:
  "Zero-Order Hold "/1 -> Real-Imag to Complex1/2
  Complex to Real-Imag/2 -> "AntiAliasing "/1
  Complex to Real-Imag/1 -> AntiAliasing/1
  In/1 -> Complex to Real-Imag/1
  Zero-Order Hold/1 -> Real-Imag to Complex1/1
  AntiAliasing/1 -> Zero-Order Hold/1
  "AntiAliasing "/1 -> "Zero-Order Hold "/1
  Real-Imag to Complex1/1 -> Out/1

== system ad9361_rx_fastattack/Test Source/Interpolation  ==
  In : Inport
  AntiAliasing : dsparch4/Analog Filter Design  method=Elliptic  filttype=Lowpass  N=8  Wlo=2*pi/(2*Tstep)  Whi=80  Rp=0.1  Rs=80
  "AntiAliasing " : dsparch4/Analog Filter Design  method=Elliptic  filttype=Lowpass  N=8  Wlo=2*pi/(2*Tstep)  Whi=80  Rp=0.1  Rs=80
  Complex to Real-Imag : ComplexToRealImag
  Real-Imag to Complex1 : RealImagToComplex
  Zero-Order Hold : ZeroOrderHold  SampleTime=Tstep/OverSample
  "Zero-Order Hold " : ZeroOrderHold  SampleTime=Tstep/OverSample
  Out : Outport
  wires:
  "Zero-Order Hold "/1 -> Real-Imag to Complex1/2
  Complex to Real-Imag/2 -> "AntiAliasing "/1
  Complex to Real-Imag/1 -> AntiAliasing/1
  In/1 -> Complex to Real-Imag/1
  Zero-Order Hold/1 -> Real-Imag to Complex1/1
  AntiAliasing/1 -> Zero-Order Hold/1
  "AntiAliasing "/1 -> "Zero-Order Hold "/1
  Real-Imag to Complex1/1 -> Out/1

== system ad9361_rx_fastattack/ADI9361_rx/ADC Overload Detector/Peak Detector ==
  In : Inport
  HTh : Constant  Value=Hthreshold  SampleTime=ad9361_rx_pars.Tadc*Ncycles
  HighThreshold : RelationalOperator  OutDataTypeStr=boolean  RndMeth=Nearest
  LTh : Constant  Value=Lthreshold  SampleTime=ad9361_rx_pars.Tadc*Ncycles
  LowThreshold : RelationalOperator  OutDataTypeStr=boolean  RndMeth=Nearest
  Out_HTh : Outport
  OutLTh : Outport  Port=2
  wires:
  LowThreshold/1 -> OutLTh/1
  HighThreshold/1 -> Out_HTh/1
  LTh/1 -> LowThreshold/2
  In/1 -> HighThreshold/1, LowThreshold/1
  HTh/1 -> HighThreshold/2

== system ad9361_rx_fastattack/ADI9361_rx/ADC Overload Detector/Peak Detector1 ==
  In : Inport
  HTh : Constant  Value=Hthreshold  SampleTime=ad9361_rx_pars.Tadc*Ncycles
  HighThreshold : RelationalOperator  OutDataTypeStr=boolean  RndMeth=Nearest
  LTh : Constant  Value=Lthreshold  SampleTime=ad9361_rx_pars.Tadc*Ncycles
  LowThreshold : RelationalOperator  OutDataTypeStr=boolean  RndMeth=Nearest
  Out_HTh : Outport
  OutLTh : Outport  Port=2
  wires:
  HTh/1 -> HighThreshold/2
  In/1 -> LowThreshold/1, HighThreshold/1
  LTh/1 -> LowThreshold/2
  HighThreshold/1 -> Out_HTh/1
  LowThreshold/1 -> OutLTh/1

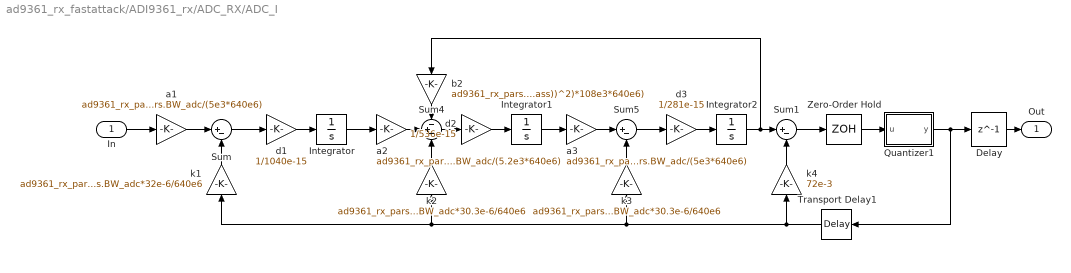
== system ad9361_rx_fastattack/ADI9361_rx/ADC_RX/ADC_I ==
  In : Inport
  Delay : Delay  DelayLength=1
  Integrator : Integrator  LimitOutput=on  UpperSaturationLimit=0.9  LowerSaturationLimit=-0.9
  Integrator1 : Integrator  LimitOutput=on  UpperSaturationLimit=0.9  LowerSaturationLimit=-0.9
  Integrator2 : Integrator  LimitOutput=on  UpperSaturationLimit=0.9  LowerSaturationLimit=-0.9
  Quantizer1 : Subsystem
  Sum : Sum  Inputs=|+-
  Sum1 : Sum  Inputs=|+-
  Sum4 : Sum  Inputs=-+-
  Sum5 : Sum  Inputs=|+-
  Transport Delay1 : TransportDelay  DelayTime=ad9361_rx_pars.Tadc/2
  Zero-Order Hold : ZeroOrderHold  SampleTime=ad9361_rx_pars.Tadc
  a1 : Gain  Gain=ad9361_rx_pars.BW_adc/(5e3*640e6)
  a2 : Gain  Gain=ad9361_rx_pars.BW_adc/(5.2e3*640e6)
  a3 : Gain  Gain=ad9361_rx_pars.BW_adc/(5e3*640e6)
  b2 : Gain  Gain=ad9361_rx_pars.BW_adc*1024/(4*((ad9361_rx_pars.BW_adc/(2*ad9361_rx_pars.Fpass))^2)*108e3*640e6)
  d1 : Gain  Gain=1/1040e-15
  d2 : Gain  Gain=1/536e-15
  d3 : Gain  Gain=1/281e-15
  k1 : Gain  Gain=ad9361_rx_pars.BW_adc*32e-6/640e6
  k2 : Gain  Gain=ad9361_rx_pars.BW_adc*30.3e-6/640e6
  k3 : Gain  Gain=ad9361_rx_pars.BW_adc*30.3e-6/640e6
  k4 : Gain  Gain=72e-3
  Out : Outport
  wires:
  k1/1 -> Sum/2
  a1/1 -> Sum/1
  Sum5/1 -> d3/1
  Sum4/1 -> d2/1
  d3/1 -> Integrator2/1
  In/1 -> a1/1
  Integrator2/1 -> Sum1/1, b2/1
  d2/1 -> Integrator1/1
  Integrator1/1 -> a3/1
  d1/1 -> Integrator/1
  Integrator/1 -> a2/1
  Sum/1 -> d1/1
  Zero-Order Hold/1 -> Quantizer1/1(u)
  a2/1 -> Sum4/2
  k2/1 -> Sum4/3
  k3/1 -> Sum5/2
  b2/1 -> Sum4/1
  a3/1 -> Sum5/1
  Sum1/1 -> Zero-Order Hold/1
  k4/1 -> Sum1/2
  Quantizer1/1(y) -> Transport Delay1/1, Delay/1
  Transport Delay1/1 -> k4/1, k1/1, k2/1, k3/1
  Delay/1 -> Out/1

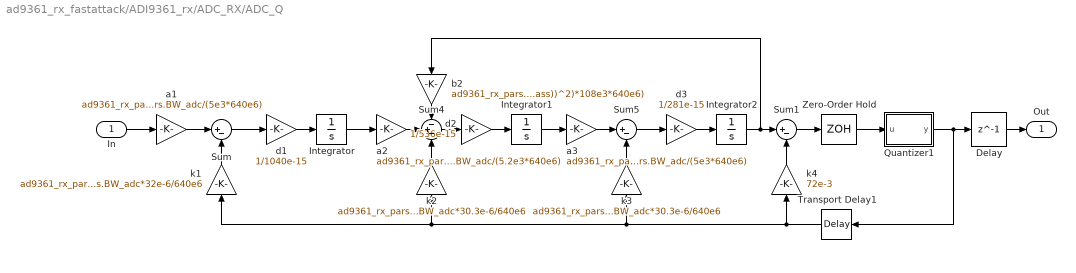
== system ad9361_rx_fastattack/ADI9361_rx/ADC_RX/ADC_Q ==
  In : Inport
  Delay : Delay  DelayLength=1
  Integrator : Integrator  LimitOutput=on  UpperSaturationLimit=0.9  LowerSaturationLimit=-0.9
  Integrator1 : Integrator  LimitOutput=on  UpperSaturationLimit=0.9  LowerSaturationLimit=-0.9
  Integrator2 : Integrator  LimitOutput=on  UpperSaturationLimit=0.9  LowerSaturationLimit=-0.9
  Quantizer1 : Subsystem
  Sum : Sum  Inputs=|+-
  Sum1 : Sum  Inputs=|+-
  Sum4 : Sum  Inputs=-+-
  Sum5 : Sum  Inputs=|+-
  Transport Delay1 : TransportDelay  DelayTime=ad9361_rx_pars.Tadc/2
  Zero-Order Hold : ZeroOrderHold  SampleTime=ad9361_rx_pars.Tadc
  a1 : Gain  Gain=ad9361_rx_pars.BW_adc/(5e3*640e6)
  a2 : Gain  Gain=ad9361_rx_pars.BW_adc/(5.2e3*640e6)
  a3 : Gain  Gain=ad9361_rx_pars.BW_adc/(5e3*640e6)
  b2 : Gain  Gain=ad9361_rx_pars.BW_adc*1024/(4*((ad9361_rx_pars.BW_adc/(2*ad9361_rx_pars.Fpass))^2)*108e3*640e6)
  d1 : Gain  Gain=1/1040e-15
  d2 : Gain  Gain=1/536e-15
  d3 : Gain  Gain=1/281e-15
  k1 : Gain  Gain=ad9361_rx_pars.BW_adc*32e-6/640e6
  k2 : Gain  Gain=ad9361_rx_pars.BW_adc*30.3e-6/640e6
  k3 : Gain  Gain=ad9361_rx_pars.BW_adc*30.3e-6/640e6
  k4 : Gain  Gain=72e-3
  Out : Outport
  wires:
  Delay/1 -> Out/1
  Transport Delay1/1 -> k3/1, k2/1, k1/1, k4/1
  Quantizer1/1(y) -> Transport Delay1/1, Delay/1
  k4/1 -> Sum1/2
  Sum1/1 -> Zero-Order Hold/1
  a3/1 -> Sum5/1
  b2/1 -> Sum4/1
  k3/1 -> Sum5/2
  k2/1 -> Sum4/3
  a2/1 -> Sum4/2
  Zero-Order Hold/1 -> Quantizer1/1(u)
  Sum/1 -> d1/1
  Integrator/1 -> a2/1
  d1/1 -> Integrator/1
  Integrator1/1 -> a3/1
  d2/1 -> Integrator1/1
  Integrator2/1 -> b2/1, Sum1/1
  In/1 -> a1/1
  d3/1 -> Integrator2/1
  Sum4/1 -> d2/1
  Sum5/1 -> d3/1
  a1/1 -> Sum/1
  k1/1 -> Sum/2

== system ad9361_rx_fastattack/ADI9361_rx/Average Power Meter/RMS ==
  In : Inport
  CountNCycles : Buffer  N=Ncycles
  Frame Conversion : FrameConversion  InheritSamplingMode=off  OutFrame=Sample-based
  Gain2 : Gain  Gain=1/Ncycles
  Root : Sqrt  SaturateOnIntegerOverflow=on
  Squared : Math  Operator=magnitude^2  SaturateOnIntegerOverflow=on
  Sum : Sum  Inputs=+
  Out : Outport
  wires:
  Sum/1 -> Gain2/1
  Frame Conversion/1 -> Out/1
  CountNCycles/1 -> Squared/1
  Squared/1 -> Sum/1
  Root/1 -> Frame Conversion/1
  Gain2/1 -> Root/1
  In/1 -> CountNCycles/1

== system ad9361_rx_fastattack/ADI9361_rx/Average Power Meter/dB Conversion ==
  in : Inport
  Constant : Constant  Value=fuzz_val  OutDataTypeStr=Inherit: Inherit via back propagation
  Constant1 : Constant  Value=dBval  OutDataTypeStr=Inherit: Inherit via back propagation
  Err if non-flt : dspsigattribs/Check Signal Attributes  SigAttribCheckMethod=Does not match attributes exactly  Complexity=Ignore  Frame=Ignore  DimsCheckMethod=Ignore  Dimensions=1-D  DatatypeCheckMethod=Is...  DatatypeGeneral=Floating-point  DtypeFloatSpecific=Any floating-point  DtypeFixedSpecific=Any fixed-point  DtypeIntSpecific=Any integer  SampleMode=Ignore
      settings: SourceProductName=DSP System Toolbox  SourceProductBaseCode=DS
  Error if Cplx : dspsigattribs/Check Signal Attributes  SigAttribCheckMethod=Matches attributes exactly  Complexity=Complex  Frame=Ignore  DimsCheckMethod=Ignore  Dimensions=1-D  DatatypeCheckMethod=Ignore  DatatypeGeneral=Boolean  DtypeFloatSpecific=Any floating-point  DtypeFixedSpecific=Any fixed-point  DtypeIntSpecific=Any integer  SampleMode=Ignore
      settings: SourceProductName=DSP System Toolbox  SourceProductBaseCode=DS
  Gain : Gain  Gain=10  SaturateOnIntegerOverflow=on  OutDataTypeStr=Inherit: Same as input  ParamDataTypeStr=Inherit: Same as input
  Magsq : Math  Operator=magnitude^2  SaturateOnIntegerOverflow=on
  Scale by R : Gain  Gain=1./R  SaturateOnIntegerOverflow=on  OutDataTypeStr=Inherit: Same as input  ParamDataTypeStr=Inherit: Same as input
  Sum1 : Sum  SaturateOnIntegerOverflow=on  InputSameDT=on  OutDataTypeStr=Inherit: Same as first input
  Sum2 : Sum  SaturateOnIntegerOverflow=on  InputSameDT=on  OutDataTypeStr=Inherit: Same as first input
  log10 : Math  Operator=log10  SaturateOnIntegerOverflow=on
  out : Outport  InitialOutput=0
  wires:
  log10/1 -> Gain/1
  Magsq/1 -> Scale by R/1
  Scale by R/1 -> log10/1
  Err if non-flt/1 -> Error if Cplx/1
  in/1 -> Err if non-flt/1
  Error if Cplx/1 -> Sum1/1
  Sum1/1 -> Magsq/1
  Constant/1 -> Sum1/2
  Gain/1 -> Sum2/1
  Sum2/1 -> out/1
  Constant1/1 -> Sum2/2

== system ad9361_rx_fastattack/ADI9361_rx/DDC_Filters_RX/Hm1 ==
  note: 1) Only subsystems can be added as variant choices at this level
      | 2) Blocks cannot be connected at this level as connectivity is
      | automatically determined at simulation, based on the active variant
  In : Inport
  Hm1 : Subsystem  VariantControl=(default)
  NoFilter : Subsystem  VariantControl=ad9361_rx_hm1Filt==0
  Out : Outport

== system ad9361_rx_fastattack/ADI9361_rx/DDC_Filters_RX/Hm2 ==
  note: 1) Only subsystems can be added as variant choices at this level
      | 2) Blocks cannot be connected at this level as connectivity is
      | automatically determined at simulation, based on the active variant
  In : Inport
  Hm2 : Subsystem  VariantControl=(default)
  NoFilter : Subsystem  VariantControl=ad9361_rx_hm2Filt==0
  Out : Outport

== system ad9361_rx_fastattack/ADI9361_rx/DDC_Filters_RX/Hm3 ==
  note: 1) Only subsystems can be added as variant choices at this level
      | 2) Blocks cannot be connected at this level as connectivity is
      | automatically determined at simulation, based on the active variant
  In : Inport
  Hm3 : Subsystem  VariantControl=(default)
  NoFilter : Subsystem  VariantControl=ad9361_rx_hm3Filt==0
  Out : Outport

== system ad9361_rx_fastattack/ADI9361_rx/DDC_Filters_RX/Hm4 ==
  note: 1) Only subsystems can be added as variant choices at this level
      | 2) Blocks cannot be connected at this level as connectivity is
      | automatically determined at simulation, based on the active variant
  In1 : Inport
  Hm4 : Subsystem  VariantControl=(default)
  NoFilter : Subsystem  VariantControl=ad9361_rx_hm4Filt==0
  Out1 : Outport

== system ad9361_rx_fastattack/ADI9361_rx/DDC_Filters_RX/dBFS ==
  In : Inport
  Complex to Real-Imag : ComplexToRealImag
  Gain3 : Gain  Gain=2047
  Quantizer : Quantizer  QuantizationInterval=1
  Quantizer1 : Quantizer  QuantizationInterval=1
  Real-Imag to Complex : RealImagToComplex
  Saturation : Saturate  UpperLimit=2047  LowerLimit=-2048
  Saturation1 : Saturate  UpperLimit=2047  LowerLimit=-2048
  Out : Outport
  wires:
  In/1 -> Gain3/1
  Quantizer/1 -> Saturation/1
  Gain3/1 -> Complex to Real-Imag/1
  Complex to Real-Imag/1 -> Quantizer1/1
  Complex to Real-Imag/2 -> Quantizer/1
  Real-Imag to Complex/1 -> Out/1
  Saturation1/1 -> Real-Imag to Complex/1
  Saturation/1 -> Real-Imag to Complex/2
  Quantizer1/1 -> Saturation1/1

== system ad9361_rx_fastattack/ADI9361_rx/LPF_RX/dB2lin ==
  In : Inport
  1/20 : Gain  Gain=1/20
  exp : Math  Operator=10^u  SaturateOnIntegerOverflow=on
  Out : Outport
  wires:
  exp/1 -> Out/1
  In/1 -> 1/20/1
  1/20/1 -> exp/1

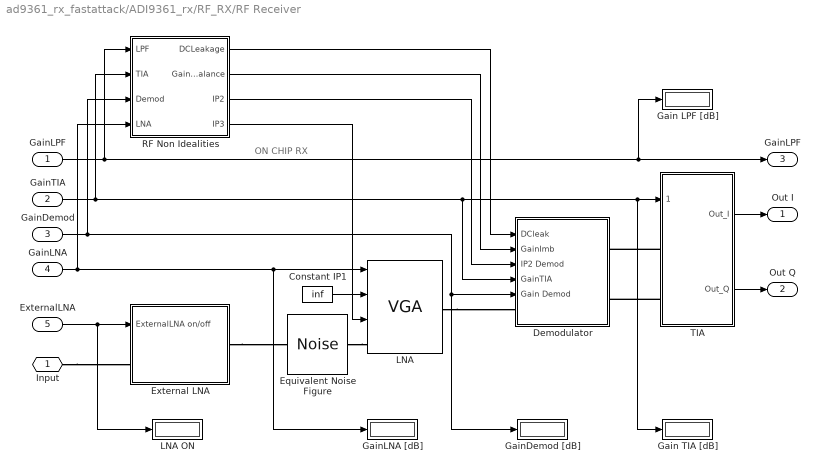
== system ad9361_rx_fastattack/ADI9361_rx/RF_RX/RF Receiver ==
  note: ON CHIP RX
  GainLPF : Inport
  GainTIA : Inport  Port=2
  GainDemod : Inport  Port=3
  GainLNA : Inport  Port=4
  ExternalLNA : Inport  Port=5
  Constant IP1 : Constant  Value=inf
  Demodulator : Subsystem
  Equivalent Noise Figure : simrfV2sources1/Noise  SimulinkInputSignalType=Ideal voltage  NoiseType=White  NoisePSD=4*1.381e-23*290*50*10^(NF/10)  CarrierFreq=fc_RF Hz  InternalGrounding=off
      settings: SourceProductName=RF Blockset  SourceProductBaseCode=RB
  External LNA : Subsystem
  Gain LPF [dB] : Display
  Gain TIA [dB] : Display
  GainDemod [dB] : Display
  GainLNA [dB] : Display
  LNA : simrfV2elements/VGA  classname=vga  Zin=Rin  Zout=50  IO=Input  InternalGrounding=on
      settings: SourceProductName=RF Blockset  SourceProductBaseCode=RB
  LNA ON : Display
  RF Non Idealities : Subsystem
  TIA : Subsystem
  Input : PMIOPort  Port=1  Side=Left
  Out I : Outport
  Out Q : Outport  Port=2
  "GainLPF " : Outport  Port=3
  wires:
  GainTIA/1 -> RF Non Idealities/2(TIA), Gain TIA [dB]/1, TIA/1(Gain TIA), Demodulator/4(GainTIA)
  TIA/1(Out_I) -> Out I/1
  TIA/2(Out_Q) -> Out Q/1
  GainDemod/1 -> RF Non Idealities/3(Demod), Demodulator/5(Gain Demod), GainDemod [dB]/1
  GainLNA/1 -> LNA/1, GainLNA [dB]/1, RF Non Idealities/4(LNA)
  GainLPF/1 -> "GainLPF "/1, Gain LPF [dB]/1, RF Non Idealities/1(LPF)
  RF Non Idealities/1(DCLeakage) -> Demodulator/1(DCleak)
  RF Non Idealities/3(IP2) -> Demodulator/3(IP2 Demod)
  RF Non Idealities/4(IP3) -> LNA/3
  Constant IP1/1 -> LNA/2
  ExternalLNA/1 -> LNA ON/1, External LNA/1(ExternalLNA on/off)
  RF Non Idealities/2(GainImbalance) -> Demodulator/2(GainImb)
  connections:
  LNA/RConn1 -- Demodulator/LConn1
  TIA/LConn1 -- Demodulator/RConn1
  TIA/LConn2 -- Demodulator/RConn2
  Equivalent Noise Figure/LConn1 -- LNA/LConn1
  Input/RConn1 -- External LNA/LConn1
  External LNA/RConn1 -- Equivalent Noise Figure/RConn1

== system ad9361_rx_fastattack/ADI9361_rx/Subsystem6/Subsystem1 ==
  Data Type Conversion : DataTypeConversion  OutDataTypeStr=boolean
  Pulse Generator2 : DiscretePulseGenerator  SampleTime=Trf
  START : Outport
  wires:
  Pulse Generator2/1 -> Data Type Conversion/1
  Data Type Conversion/1 -> START/1

== system ad9361_rx_fastattack/ADI9361_rx/Subsystem6/Wblk5 ==
  Win : Inport
  Sin : Inport  Port=2
  Combinatorial Logic : CombinatorialLogic  TruthTable=[0; 0; 1; 0]
  Mux : Mux  Inputs=2
  Wout : Outport
  wires:
  Mux/1 -> Combinatorial Logic/1
  Combinatorial Logic/1 -> Wout/1  "wout"
  Win/1 -> Mux/1
  Sin/1 -> Mux/2

== system ad9361_rx_fastattack/ADI9361_rx/Subsystem6/Wblk6 ==
  Win : Inport
  Sin : Inport  Port=2
  Combinatorial Logic : CombinatorialLogic  TruthTable=[0; 0; 1; 0]
  Mux : Mux  Inputs=2
  Wout : Outport
  wires:
  Mux/1 -> Combinatorial Logic/1
  Combinatorial Logic/1 -> Wout/1  "wout"
  Win/1 -> Mux/1
  Sin/1 -> Mux/2

== system ad9361_rx_fastattack/ADI9361_rx/Subsystem6/Wblk7 ==
  Win : Inport
  Sin : Inport  Port=2
  Combinatorial Logic : CombinatorialLogic  TruthTable=[0; 0; 1; 0]
  Mux : Mux  Inputs=2
  Wout : Outport
  wires:
  Mux/1 -> Combinatorial Logic/1
  Combinatorial Logic/1 -> Wout/1  "wout"
  Win/1 -> Mux/1
  Sin/1 -> Mux/2

== system ad9361_rx_fastattack/ADI9361_rx/ADC_RX/ADC_I/Quantizer1 ==
  u : Inport
  Abs : Abs
  Idealized ADC quantizer : simulink_extras/Additional Discrete/Idealized ADC quantizer  NumberOfConverterBits=3  Vmin=0  Vmax=.8  OutputDataType=double  OutputNegativeValues=off
      settings: SourceProductName=Simulink
  Product : Product
  Saturation : Saturate  UpperLimit=0.41
  Sign : Signum
  y : Outport
  wires:
  u/1 -> Sign/1, Abs/1
  Saturation/1 -> Idealized ADC quantizer/1
  Idealized ADC quantizer/1 -> Product/1
  Sign/1 -> Product/2
  Abs/1 -> Saturation/1
  Product/1 -> y/1
